simulink model "FIR_filter"  (R2020b)
settings: Solver=FixedStepAuto  StartTime=0.0  StopTime=10.0  FixedStep=0.2  RelTol=1e-3
settings Model: Creator=omkar  LastModifiedBy=omkar
settings DataIOCC: SaveOutput=off  SaveTime=off

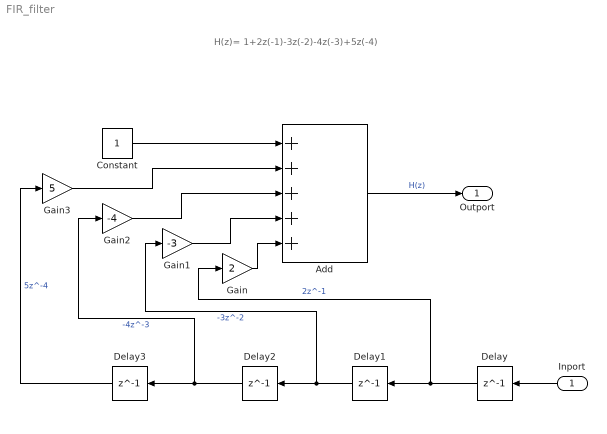
== system FIR_filter ==
  note: H(z)= 1+2z(-1)-3z(-2)-4z(-3)+5z(-4)
  Inport : Inport  OutDataTypeStr=double  PortDimensions=1
  Add : Sum  Inputs=+++++
  Constant : Constant
  Delay{,1..3} (4 alike) : Delay  DelayLength=1
  Gain : Gain  Gain=2
  Gain1 : Gain  Gain=-3
  Gain2 : Gain  Gain=-4
  Gain3 : Gain  Gain=5
  Outport : Outport  OutDataTypeStr=double  PortDimensions=1  SampleTime=[0.20000000000000001,0]
  wires:
  Delay3/1 -> Gain3/1  "5z^-4"
  Delay2/1 -> Gain2/1, Delay3/1  "-4z^-3"
  Delay1/1 -> Gain1/1, Delay2/1  "-3z^-2"
  Delay/1 -> Gain/1, Delay1/1  "2z^-1"
  Gain3/1 -> Add/2
  Gain2/1 -> Add/3
  Inport/1 -> Delay/1
  Gain1/1 -> Add/4
  Gain/1 -> Add/5
  Add/1 -> Outport/1  "H(z)"
  Constant/1 -> Add/1
